simulink model "sl_ctorque"  (Simulink 7.7)
settings: Solver=ode45  StartTime=0.0  StopTime=10  FixedStep=0.01  MaxStep=0.05  RelTol=1e-3
PreLoadFcn:
  | puma560
  | p560 = nofriction(p560);
libraries: roblocks x4
settings Model: Creator=pic  LastModifiedBy=corkep  ExtModeTrigMode=oneshot  ExtModeArmWhenConnect=off
settings SolverCC: ZeroCrossControl=DisableAll
settings DataIOCC: LimitDataPoints=off  ReturnWorkspaceOutputs=on
settings OptimizationCC: BlockReduction=off  BooleanDataType=off  InitFltsAndDblsToZero=on
settings DebuggingCC: SaveWithParameterizedLinksMsg=none  SignalResolutionControl=TryResolveAllWithWarning  SolverPrmCheckMsg=none  MultiTaskDSMMsg=warning  MultiTaskCondExecSysMsg=none  StrictBusMsg=None
settings HardwareCC: TargetUnknown=on
settings RTWCC: IncludeERTFirstTime=on
settings GRTTargetCC: ModelReferenceCompliant=off  CompOptLevelCompliant=off  MatFileLogging=off

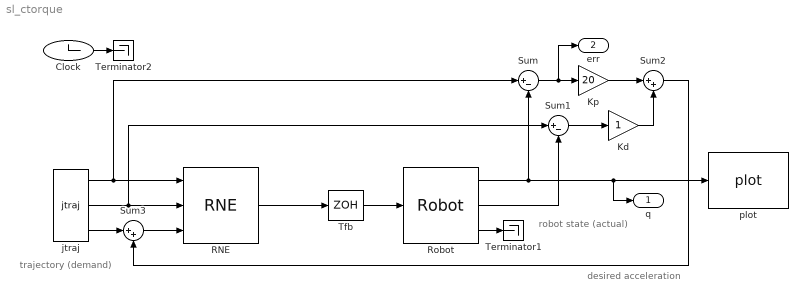
== system sl_ctorque ==
  note: trajectory
      | (demand)
  note: robot state
      | (actual)
  note: desired acceleration
  Clock : Clock
      settings: Decimation=10
  Kd : Gain  SaturateOnIntegerOverflow=on  OutDataTypeStr=Inherit: Same as input  ParamDataTypeStr=Inherit: Same as input
  Kp : Gain  Gain=20  SaturateOnIntegerOverflow=on  OutDataTypeStr=Inherit: Same as input  ParamDataTypeStr=Inherit: Same as input
  RNE : roblocks/Dynamics/RNE  SystemSampleTime=-1  robot=p560.nofriction()  grav=[0 0 9.81]
  Robot : roblocks/Dynamics/Robot  SystemSampleTime=-1  robot=p560.nofriction()  q0=[0 0 0 0 0 0]
  Sum : Sum  Inputs=|+-  SaturateOnIntegerOverflow=on  InputSameDT=on  OutDataTypeStr=Inherit: Same as first input
  Sum1 : Sum  Inputs=|+-  SaturateOnIntegerOverflow=on  InputSameDT=on  OutDataTypeStr=Inherit: Same as first input
  Sum2 : Sum  Inputs=|++  SaturateOnIntegerOverflow=on  InputSameDT=on  OutDataTypeStr=Inherit: Same as first input
  Sum3 : Sum  Inputs=|++  SaturateOnIntegerOverflow=on  InputSameDT=on  OutDataTypeStr=Inherit: Same as first input
  Terminator1 : Terminator
  Terminator2 : Terminator
  Tfb : ZeroOrderHold  SampleTime=0.01
  jtraj : roblocks/Trajectory/jtraj  SystemSampleTime=-1  q0=[0 0 0 0 0 0]  qf=[pi/4 pi/2 -pi/2 0 0 0]  tmax=10  ts=-1
  plot : roblocks/Robot Graphics/plot  SystemSampleTime=-1  robot=p560  fps=25
  q : Outport
  err : Outport  Port=2
  wires:
  Sum/1 -> Kp/1, err/1
  Kp/1 -> Sum2/1
  Robot/1 -> Sum/2, q/1, plot/1
  Robot/2 -> Sum1/2
  RNE/1 -> Tfb/1
  jtraj/1 -> Sum/1, RNE/1
  jtraj/2 -> Sum1/1, RNE/2
  Sum1/1 -> Kd/1
  Kd/1 -> Sum2/2
  jtraj/3 -> Sum3/1
  Robot/3 -> Terminator1/1
  Clock/1 -> Terminator2/1
  Sum3/1 -> RNE/3
  Sum2/1 -> Sum3/2
  Tfb/1 -> Robot/1
